simulink model "corr_mod_1_sim41_MI"  (R2019b)
settings: Solver=ode5  StartTime=0  StopTime=1  FixedStep=0.001  MaxStep=0.01  RelTol=1e-3  AbsTol=1e-3
undefined symbols (not defined in the file): g, l, m, M
settings Model: ExtModeTrigMode=oneshot  ExtModeArmWhenConnect=off  ExtModeAutoUpdateStatusClock=off  Creator=franckplestan  LastModifiedBy=15043
settings SolverCC: AutoScaleAbsTol=off
settings DataIOCC: SaveFormat=Array  SignalLoggingSaveFormat=ModelDataLogs  SaveOutput=off  ReturnWorkspaceOutputs=off
settings OptimizationCC: BooleanDataType=off  ExpressionDepthLimit=2147483647  InitFltsAndDblsToZero=on  LifeSpan=inf
settings DebuggingCC: SaveWithParameterizedLinksMsg=none  UnderspecifiedInitializationDetection=Classic  MergeDetectMultiDrivingBlocksExec=none  SignalResolutionControl=TryResolveAllWithWarning  MultiTaskDSMMsg=warning  MultiTaskCondExecSysMsg=none  FcnCallInpInsideContextMsg=warning  StateNameClashWarn=warning  SFUnexpectedBacktrackingDiag=warning  SFNoUnconditionalDefaultTransitionDiag=warning  SFExecutionAtInitializationDiag=none  ArithmeticOperatorsInVariantConditions=warning
settings HardwareCC: ProdBitPerPointer=32  ProdBitPerSizeT=32  ProdBitPerPtrDiffT=32  ProdLargestAtomicFloat=None  ProdIntDivRoundTo=Undefined  ProdEndianess=Unspecified  ProdWordSize=32  ProdHWDeviceType=32-bit Generic  TargetUnknown=on
settings ModelReferenceCC: PropagateSignalLabelsOutOfModel=off
settings SFSimCC: SimUseLocalCustomCode=off  CustomCodeUndefinedFunction=UseInterfaceOnly
settings RTWCC: RTWUseLocalCustomCode=off
settings CodeAppCC: StateflowObjectComments=on
settings GRTTargetCC: TargetLangStandard=C89/C90 (ANSI)  ModelReferenceCompliant=off  ParMdlRefBuildCompliant=off  CompOptLevelCompliant=off  ConcurrentExecutionCompliant=off  GeneratePreprocessorConditionals=Disable all  CombineOutputUpdateFcns=off  MatFileLogging=off  MATLABClassNameForMDSCustomization=Simulink.SoftwareTarget.TargetSpecificTriggerConfigurationBase  GRTInterface=on
settings ConfigComp: CovMetricSettings=dw  CovHtmlReporting=on  CovSaveCumulativeToWorkspaceVar=on  CovSaveSingleToWorkspaceVar=on  CovExternalEMLEnable=off  CovSFcnEnable=off

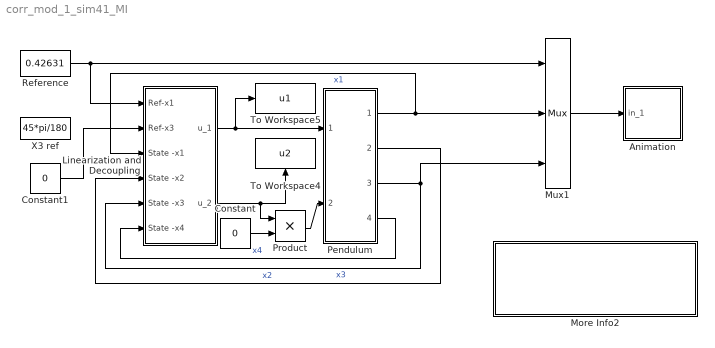
== system corr_mod_1_sim41_MI ==
  Animation : Subsystem  mask(Pendulum plot){RefBlock=Reference}
      mask prompts: RefBlock "DC reference signal block name:"
      mask help: Pendulum plot
      mask Help: Pendulum animation function using Handle graphics.
      mask Display: plot([-10 10],[0 0],[-2 -2 2 2],[0 1 1 0],[0 3],[1 5])
  Constant : Constant  Value=0
  Constant1 : Constant  Value=0
  Linearization and Decoupling : Subsystem
  More Info2 : Subsystem
      settings: OpenFcn=cipendco
      mask Display: disp('Init-File cipendco-doubleclick')
  Mux1 : Mux  Inputs=3
  Pendulum : Subsystem
  Product : Product
  Reference : Constant  Value=0.42631
  To Workspace4 : ToWorkspace  VariableName=u2  SampleTime=-1
  To Workspace5 : ToWorkspace  VariableName=u1  SampleTime=-1
  X3 ref : Constant  Value=45*pi/180
  wires:
  Pendulum/2(State-x2) -> Linearization and Decoupling/4(State -x2)  "x2"
  Pendulum/4(State-x4) -> Linearization and Decoupling/6(State -x4)  "x4"
  Linearization and Decoupling/2(u_2) -> Product/1, To Workspace4/1
  Mux1/1 -> Animation/1(in_1)
  Pendulum/3(State-x3) -> Linearization and Decoupling/5(State -x3), Mux1/3  "x3"
  Reference/1 -> Linearization and Decoupling/1(Ref-x1), Mux1/1
  Pendulum/1(State-x1) -> Linearization and Decoupling/3(State -x1), Mux1/2  "x1"
  Linearization and Decoupling/1(u_1) -> Pendulum/1(Input-u1), To Workspace5/1
  Constant/1 -> Product/2
  Product/1 -> Pendulum/2(Unput-u2)
  Constant1/1 -> Linearization and Decoupling/2(Ref-x3)

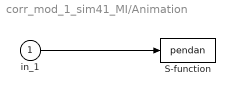
== system corr_mod_1_sim41_MI/Animation ==
  in_1 : Inport
  S-function : S-Function  FunctionName=pendan  Parameters=RefBlock  SFunctionDeploymentMode=off  EnableBusSupport=off
      settings: DeleteFcn=pendan([],[],[],'DeleteBlock');
  wires:
  in_1/1 -> S-function/1

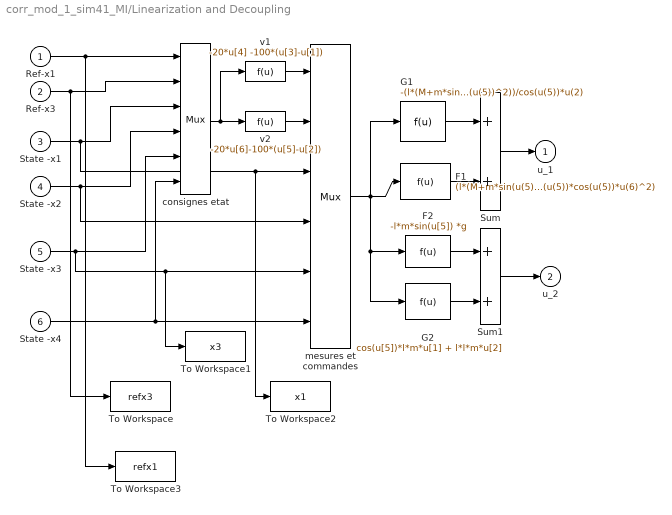
== system corr_mod_1_sim41_MI/Linearization and Decoupling ==
  Ref-x1 : Inport
  Ref-x3 : Inport  Port=2
  State -x1 : Inport  Port=3
  State -x2 : Inport  Port=4
  State -x3 : Inport  Port=5
  State -x4 : Inport  Port=6
  F1 : Fcn  Expr=(l*(M+m*sin(u(5))^2))/cos(u(5))*((M+m)*g*sin(u(5))+m*l*sin(u(5))*cos(u(5))*u(6)^2)
  F2 : Fcn  Expr=-l*m*sin(u[5]) *g
  G1 : Fcn  Expr=-(l*(M+m*sin(u(5))^2))/cos(u(5))*u(2)
  G2 : Fcn  Expr=cos(u[5])*l*m*u[1] + l*l*m*u[2]
  Sum : Sum  SaturateOnIntegerOverflow=on  InputSameDT=on  OutDataTypeStr=Inherit: Same as first input
  Sum1 : Sum  SaturateOnIntegerOverflow=on  InputSameDT=on  OutDataTypeStr=Inherit: Same as first input
  To Workspace : ToWorkspace  VariableName=refx3  SampleTime=-1
  To Workspace1 : ToWorkspace  VariableName=x3  SampleTime=-1
  To Workspace2 : ToWorkspace  VariableName=x1  SampleTime=-1
  To Workspace3 : ToWorkspace  VariableName=refx1  SampleTime=-1
  consignes etat : Mux  Inputs=6
  mesures et commandes : Mux  Inputs=6
  v1 : Fcn  Expr=-20*u[4] -100*(u[3]-u[1])
  v2 : Fcn  Expr=-20*u[6]-100*(u[5]-u[2])
  u_1 : Outport  VectorParamsAs1DForOutWhenUnconnected=off
  u_2 : Outport  Port=2  VectorParamsAs1DForOutWhenUnconnected=off
  wires:
  F1/1 -> Sum/2
  F2/1 -> Sum1/1
  G2/1 -> Sum1/2
  G1/1 -> Sum/1
  v1/1 -> mesures et commandes/1
  v2/1 -> mesures et commandes/2
  mesures et commandes/1 -> G1/1, F2/1, G2/1, F1/1
  consignes etat/1 -> v1/1, v2/1
  State -x3/1 -> consignes etat/5, mesures et commandes/5, To Workspace1/1
  State -x2/1 -> consignes etat/4, mesures et commandes/4
  State -x1/1 -> consignes etat/3, mesures et commandes/3, To Workspace2/1
  State -x4/1 -> consignes etat/6, mesures et commandes/6
  Ref-x3/1 -> consignes etat/2, To Workspace/1
  Ref-x1/1 -> consignes etat/1, To Workspace3/1
  Sum1/1 -> u_2/1
  Sum/1 -> u_1/1

== system corr_mod_1_sim41_MI/More Info2 ==

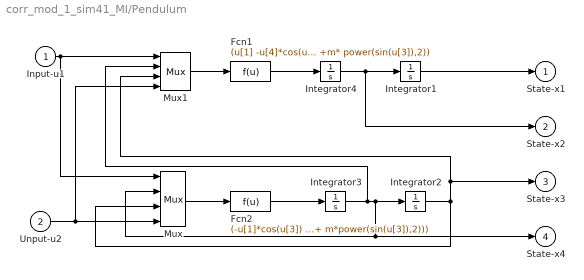
== system corr_mod_1_sim41_MI/Pendulum ==
  Input-u1 : Inport
  Unput-u2 : Inport  Port=2
  Fcn1 : Fcn  Expr=(u[1] -u[4]*cos(u[3])/l- m*g*sin(u[3])*cos(u[3]) + m*l*power(u[2],2)*sin(u[3]))/(M +m* power(sin(u[3]),2))
  Fcn2 : Fcn  Expr=(-u[1]*cos(u[3]) + u[4]*(M+m)/(m*l) + (M+m)*g*sin(u[3]) - m*l*power(u[2],2)*sin(u[3])*cos(u[3]))/(l*(M + m*power(sin(u[3]),2)))
  Integrator1 : Integrator
  Integrator2 : Integrator  InitialCondition=0.5
  Integrator3 : Integrator
  Integrator4 : Integrator
  Mux : Mux
  Mux1 : Mux
  State-x1 : Outport  VectorParamsAs1DForOutWhenUnconnected=off
  State-x2 : Outport  Port=2  VectorParamsAs1DForOutWhenUnconnected=off
  State-x3 : Outport  Port=3  VectorParamsAs1DForOutWhenUnconnected=off
  State-x4 : Outport  Port=4  VectorParamsAs1DForOutWhenUnconnected=off
  wires:
  Integrator2/1 -> Mux/3, Mux1/3, State-x3/1
  Input-u1/1 -> Mux1/1, Mux/1
  Integrator3/1 -> Integrator2/1, Mux/2, State-x4/1, Mux1/2
  Fcn1/1 -> Integrator4/1
  Mux1/1 -> Fcn1/1
  Mux/1 -> Fcn2/1
  Fcn2/1 -> Integrator3/1
  Unput-u2/1 -> Mux/4, Mux1/4
  Integrator1/1 -> State-x1/1
  Integrator4/1 -> Integrator1/1, State-x2/1
